simulink model "FILTRO_POTENTE"  (R2020a)
settings: Solver=VariableStepAuto  StartTime=0.0  StopTime=500  RelTol=1e-3
values from neighbouring files (symbols this model uses):
  distanceFromWall = 8    [missionC.m]
  nav_DT = 0.1    [initialization_nav.m]
  nav_giro = 2    [initialization_nav.m]
  nav_h0 = 0    [initialization_nav.m]
  nav_lat0 = cornerC(1)    [initialization_nav.m]
  nav_lon0 = cornerC(2)    [initialization_nav.m]
  nav_plane_AB = coefficient_plane(nav_A,nav_B)    [initialization_nav.m]
  nav_plane_BC = coefficient_plane(nav_B,nav_C)    [initialization_nav.m]
  nav_plane_CD = coefficient_plane(nav_C,nav_D)    [initialization_nav.m]
  nav_plane_DA = coefficient_plane(nav_D,nav_A)    [initialization_nav.m]
undefined symbols (not defined in the file or in its folder): nav_A, nav_B, nav_C, nav_D
(part 3 of 3)

== matlab function FILTRO_POTENTE/Navigation2/Extended Kalman Filter/MISURA VIRTUALE/MATLAB Function ==
  data: x_k_k_1 input; flag_vect input; mis_vect input; e output size=6 1; H output size=6 3; J input; nav_plane_AB parameter; nav_plane_BC parameter; nav_plane_CD parameter; nav_plane_DA parameter
%%
% chiedere ai sensoristi se le posizioni dei sensori equivalgono al centro
% di massa del robot o dobbiamo considerare spostamenti e orientazioni
% relative alla terna body
%%

function [e, H] = virtual(x_k_k_1, flag_vect, mis_vect, J, nav_plane_AB, nav_plane_BC, nav_plane_CD, nav_plane_DA)

    e = zeros(6,1);
    h = zeros(6,1);
    z = zeros(6,1);
    H = zeros(6,3);
    
    
    %valutazione misure GPS
    if mis_vect(3)==1                                   %se i dati del GPS sono validi
        if flag_vect(1) == 1 && flag_vect(2) == 1       %se i dati del GPS sono nuovi
            
            z = z + [mis_vect(1) mis_vect(2) 0 0 0 0]';
            h = h + [x_k_k_1(1)   x_k_k_1(2) 0 0 0 0]';
        
            H(1,:)= [1 0 0];
            H(2,:)= [0 1 0];
        end
    end
    
    %valutazione misure depth
    if flag_vect(4) == 1                                 %se i dati del profondimetro sono nuovi
            
        z = z + [0 0 mis_vect(4) 0 0 0]'; 
        h = h + [0 0  x_k_k_1(3) 0 0 0]';

        H(3,:)= [0 0 1];
    end
    
    %valutiamo ora le misure virtuali solo se quelle del GPS non sono
    %valide
    if mis_vect(3)==0                      %se i dati del GPS non sono validi
        
        if flag_vect(5) == 1               %se i dati del sonar di prua sono nuovi
                
                versore_son_NED = J*[1 0 0]';          %versore terna NED sonar prua
                
                [distanza, plane] = inter(x_k_k_1, versore_son_NED ,nav_plane_AB,nav_plane_BC,nav_plane_CD,nav_plane_DA);
                z = z + [0 0 0 mis_vect(5) 0 0]'; 
                h = h + [0 0 0 distanza    0 0]';
                
                H_new=zeros(1,3);
                [H_new(1), H_new(2), H_new(3)] = calc_H_vect(x_k_k_1, versore_son_NED,plane);
                H(4,:) = H_new;                
        end
    
        if flag_vect(6) == 1               %se i dati del sonar destro sono nuovi
                
                versore_son_NED = J*[0 1 0]';          %versore terna NED sonar dx
                
                [distanza, plane] = inter(x_k_k_1, versore_son_NED ,nav_plane_AB,nav_plane_BC,nav_plane_CD,nav_plane_DA);
                z = z + [0 0 0 0 mis_vect(6) 0]'; 
                h = h + [0 0 0 0 distanza    0]';
                
                H_new=zeros(1,3);
                [H_new(1), H_new(2), H_new(3)] = calc_H_vect(x_k_k_1, versore_son_NED,plane);
                H(5,:) = H_new;
        end
    
        if flag_vect(7) == 1               %se i dati del sonar sinistro sono nuovi
                 
                versore_son_NED = J*[0 -1 0]';          %versore terna NED sonar sx
                
                [distanza, plane] = inter(x_k_k_1, versore_son_NED ,nav_plane_AB,nav_plane_BC,nav_plane_CD,nav_plane_DA);
                z = z + [0 0 0 0 0 mis_vect(7)]'; 
                h = h + [0 0 0 0 0 distanza   ]'; 
                
                H_new=zeros(1,3);
                [H_new(1), H_new(2), H_new(3)] = calc_H_vect(x_k_k_1, versore_son_NED,plane);
                H(6,:) = H_new;
        end
    end
    
    e = z - h;
    
    %%riduco le dimensioni della matrice H e del vettore e
    
    i=0;
    if mis_vect(3) == 0                    %se i dati del GPS non sono validi
        H(1-i,:) = [];
        e(1-i) = [];
        i=i+1;
        H(2-i,:) = [];
        e(2-i) = [];
        i=i+1;
        if flag_vect(4) == 0               %se i dati del profondimetro non sono nuovi
            H(3-i,:) = [];
            e(3-i) = [];
            i=i+1;
        end
        if flag_vect(5) == 0               %se i dati del sonar di prua non sono nuovi
            H(4-i,:) = [];
            e(4-i) = [];
            i=i+1;
        end
        if flag_vect(6) == 0               %se i dati del sonar sinistro non sono nuovi
            H(5-i,:) = [];
            e(5-i) = [];
            i=i+1;
        end
        if flag_vect(7) == 0               %se i dati del sonar destro non sono nuovi
            H(6-i,:) = [];
            e(6-i) = [];
        end
    % da qui invece abbiamo il GPS valido
    else
        if flag_vect(1)==0 || flag_vect(2)==0  %se i dati del GPS non sono nuovi
            H(1-i,:) = [];
            e(1-i) = [];
            i=i+1;
            H(2-i,:) = [];
            e(2-i) = [];
            i=i+1;
        end
        
        if flag_vect(4) == 0               %se i dati del profondimetro non sono nuovi
            H(3-i,:) = [];
            e(3-i) = [];
            i=i+1;
        end
        
        H(4-i,:) = [];                      %annulliamo le misure dei sonar
        e(4-i) = [];
        i=i+1;
        H(5-i,:) = [];
        e(5-i) = [];
        i=i+1;
        H(6-i,:) = [];        
        e(6-i) = [];    
    end
    i=0;
end



%%
%%%%%%%%%%%%%%%%%%%%%%%%%%%%%%%%%%%%%%%%%%%%%%%%%%%%%%%%%%%%%%%%%%%%%%%%%%%%%%%%%%%%%%%%

function [dist, plane] = inter(pos, versore_son_NED,nav_plane_AB,nav_plane_BC,nav_plane_CD,nav_plane_DA)
    
    %calcolo della distanza dalla posizione ai piani delle pareti seguendo
    %la direzione data dal versore del sonar

    t_AB = -(pos(1)+nav_plane_AB(2)*pos(2)+nav_plane_AB(4))/(nav_plane_AB(2)*versore_son_NED(2)+versore_son_NED(1));
    t_BC = -(pos(1)+nav_plane_BC(2)*pos(2)+nav_plane_BC(4))/(nav_plane_BC(2)*versore_son_NED(2)+versore_son_NED(1));
    t_CD = -(pos(1)+nav_plane_CD(2)*pos(2)+nav_plane_CD(4))/(nav_plane_CD(2)*versore_son_NED(2)+versore_son_NED(1));
    t_DA = -(pos(1)+nav_plane_DA(2)*pos(2)+nav_plane_DA(4))/(nav_plane_DA(2)*versore_son_NED(2)+versore_son_NED(1));
    
    if t_AB < 0
        t_AB = inf;
    end
    if t_BC < 0
        t_BC = inf;
    end
    if t_CD < 0
        t_CD = inf;
    end
    if t_DA < 0
        t_DA = inf;
    end
           
    [dist, index] = min([t_AB t_BC t_CD t_DA]);
    dist = dist - 0.267;       %va tolto il raggio del robot rispetto al centro di massa
    
    switch index
        case 1
            plane = nav_plane_AB;
        case 2
            plane = nav_plane_BC;
        case 3
            plane = nav_plane_CD;
        case 4
            plane = nav_plane_DA;
        otherwise
            plane=[0 0 0 0];
            disp('errore nella intersezione del piano')
    end
    
end

function [H1, H2, H3]= calc_H_vect(pos, sonar, plane)

    H1 = sign(pos(1) + plane(4) + pos(2)*plane(2))/abs(sonar(1) + plane(2)*sonar(2));
    H2 = (plane(2)*sign(pos(1) + plane(4) + pos(2)*plane(2)))/abs(sonar(1) + plane(2)*sonar(2));   
    H3 = 0;
end

== matlab function FILTRO_POTENTE/Navigation2/Extended Kalman Filter/PREDIZIONE/Passo di Predizione ==
  data: x0 input; P0 input; x_k_1 input; u_k_1 input; x_k output; P_k_1 input; P_k output size=3 3; J input; L input; Q_k_1 input; nav_DT parameter; nav_flag_init input; nav_flag_init output
%% Passo di PREDIZIONE

function [x_k,  P_k, nav_flag_init] = prediction(x0, P0, x_k_1, u_k_1,  P_k_1, J, L, Q_k_1, nav_DT, nav_flag_init)
    
    x_k = zeros(3,1);
    P_k = zeros(3,3);

    % il valore di nav_flag_init è all'inizio della simulazione pari a 0
    % appena c'è il primo dato disponibile del GPS (insieme al profondimetro)
    % si assume quella come punto di inizializzazione del filtro.

    if nav_flag_init ~= 0      
        if nav_flag_init == 1
            x_k_1 = x0;
            P_k_1 = P0;
            nav_flag_init = 2;      % =2 così l'inizializzazione è fatta una sola volta.
        end
        
        %passo di predizione       
        x_k = x_k_1 + nav_DT*J*u_k_1;
        P_k = P_k_1 + L*Q_k_1*L';               %la matrice F è F = I
           
    end
end

== matlab function FILTRO_POTENTE/Navigation2/Extended Kalman Filter/Q_error/MATLAB Function4 ==
  data: Q input; Q_k_1 input; Q_k output; flag_AHRS input; flag_DVL input
function Q_k = fcn(Q, Q_k_1, flag_AHRS, flag_DVL)

    Q_k = Q;
    
    K=10;
    if flag_DVL == 1
       Q_k = Q_k_1 + K*diag([0,0,0,(0.012)^2,(0.012)^2,(0.012)^2]);
    end
    
    if flag_AHRS == 1
       Q_k = Q_k_1 + K*diag([0.0087, 0.0087, 0.0017,0,0,0]);  
    end
        
end

== matlab function FILTRO_POTENTE/Navigation2/Gyro_check/MATLAB Function4 ==
  data: flag_gyro output; gyro_new input; gyro_now output; gyro_old input
function [flag_gyro, gyro_now] = fcn(gyro_new, gyro_old)

    if isnan(gyro_new(1,1)) || isnan(gyro_new(2,1)) || isnan(gyro_new(3,1))
        gyro_now = gyro_old;
        flag_gyro = 1;
        disp('Misura gyro non valida')
    else
        gyro_now = gyro_new;
        flag_gyro = 0;
    end  
end

== matlab function FILTRO_POTENTE/Navigation2/MATLAB Function ==
  data: u input; y output
function y = Wrap2pi(u)
y = [0;0;0];
coder.extrinsic('wrapToPi');
y = wrapToPi(u);
end

== matlab function FILTRO_POTENTE/Navigation2/MATLAB Function1 ==
  data: u input; dev_standard_xy output; dev_standard_z output
function [dev_standard_xy,dev_standard_z] = fcn(u) 
    
    dev_standard_xy = sqrt(u(1,1)+u(2,2));
    dev_standard_z = sqrt(u(3,3));

end

== matlab function FILTRO_POTENTE/Navigation2/NED2ECEF ==
  data: pos_es_NED input; pos_es_ECEF output; nav_lat0 parameter; nav_lon0 parameter; nav_h0 parameter


function pos_es_ECEF = pos_NED2ECEF(pos_es_NED,nav_lat0, nav_lon0, nav_h0)
     
    coder.extrinsic('evalin', 'wgs84Ellipsoid', 'ned2geodetic');
    pos_es_ECEF = zeros(3,1);
    depth = pos_es_NED(3); 
    
    [pos_es_ECEF(1),pos_es_ECEF(2),pos_es_ECEF(3)]= ned2geodetic(pos_es_NED(1),pos_es_NED(2),0,nav_lat0,nav_lon0,nav_h0,wgs84Ellipsoid);
    pos_es_ECEF(3) = depth;
end

== matlab function FILTRO_POTENTE/Navigation2/SOS_flag_generator/MATLAB Function ==
  data: P_es input; SOS output; DVL input; AHRS input; gyro input; contatore input size=3 1; contatore output
%% Generazione flag di emergenza
% 1. Assenza di segnali dai sensori per un determinato tempo

function [SOS, contatore] = SOS_flag(P_es, DVL, AHRS, gyro, contatore)
    SOS=0;
 
    soglia_P = 10; %[m^2]
    if P_es(1,1)+P_es(2,2) > soglia_P || P_es(3,3) > soglia_P
        SOS=1;
    end
    
    if DVL == 1 
        contatore(1) = contatore(1) + 1;
    else
        contatore(1) = 0;
    end
    
    if AHRS == 1 
        contatore(2) = contatore(2) + 1;
    else
        contatore(2) = 0;
    end
    
    if gyro == 1 
        contatore(3) = contatore(3) + 1;
    else
        contatore(3) = 0;
    end
    
    if max(contatore) > 20
        SOS=1;
    end
    
    

end

== matlab function FILTRO_POTENTE/Navigation1/ECEF2NED ==
  data: GPS_ECEF input; GPS_NED output; nav_lat0 parameter; nav_lon0 parameter; nav_h0 parameter
%Componente di ingresso in terna ECEF
%Lat  [gradi]
%Long  [gradi]
%flag data_valid

function GPS_NED = GPS_conv_valid(GPS_ECEF, nav_lat0, nav_lon0, nav_h0)
    
    coder.extrinsic('evalin', 'wgs84Ellipsoid', 'geodetic2ned');

    if GPS_ECEF(3)==1
        GPS_NED = zeros(3,1);
        [GPS_NED(1),GPS_NED(2),GPS_NED(3)]= geodetic2ned(GPS_ECEF(1),GPS_ECEF(2),0,nav_lat0,nav_lon0,nav_h0,wgs84Ellipsoid);
        GPS_NED(3) = GPS_ECEF(3);
    else                            %qui ci risparmiamo la conversione se il dato non è valido
        GPS_NED = GPS_ECEF; 
    end
end

== matlab function FILTRO_POTENTE/Navigation1/Extended Kalman Filter/CORREZIONE/MATLAB Function ==
  data: x_k_k_1 input; x_k output; P_k_k_1 input; e input size=6 1; H input size=6 3; R_k input size=6 6; P_k output; nav_flag_init input


function [x_k, P_k] = correction(x_k_k_1,P_k_k_1, e, H, R_k,nav_flag_init)
    
     x_k = zeros(3,1);
     P_k = zeros(3,3);
     
     
    if nav_flag_init ~= 0
        %matrice ottenuta da derivata di funzione h (6x1) per i rumori sei vari
        %sensori, che sono 6. (ha dimensione 6x6)
        %andrebbero anche considerati i rumori legati all'AHRS che al momento
        %sono trascurati
        %M = eye(6,6);              %M è l'dientità
        S_k = H*P_k_k_1*H'+ R_k;
        K_k = P_k_k_1*H'*(inv(S_k));

        P_k = (eye(3)-(K_k*H))*P_k_k_1;
        x_k = x_k_k_1 + K_k * e;
    end

end

== matlab function FILTRO_POTENTE/MATLAB Function ==
  data: u input; y output
function y = fcn(u)
u(3)=1;
y = u;

== matlab function FILTRO_POTENTE/Navigation1/Extended Kalman Filter/Creazione vettore delle misure ==
  data: flag_vect output; GPS input; mis_vect output; depth input; s_pr input; s_dx input; s_sx input; mis_vect_prec input; J input; pos input; nav_plane_AB parameter; nav_plane_BC parameter; nav_plane_CD parameter; nav_plane_DA parameter; nav_A parameter; nav_B parameter; nav_C parameter; nav_D parameter; distanceFromWall parameter
%%
% Questa funzione impila le informazioni derivanti dai vari sensori in un
% unico vettore mis_vect 7x1.                                 
% Ci sarà un corrispondente vettore flag_vect 7x1 di flag che sarà pari a:

% flag(i) = 0  se la misura è uguale a quella arrivata nell'istante
% predecente, in tal caso la correzione non verrà effettuata
% flag(i) = 1 se la misura è stata aggiornata rispetto a quella precendente
 
% NB il controllo sulla validità dei dati del GPS è valutata nel blocco
% sucessivo

function [flag_vect,mis_vect] = misure_vector(GPS,depth,s_pr,s_dx,s_sx, mis_vect_prec,...
          J,pos, nav_plane_AB, nav_plane_BC, nav_plane_CD, nav_plane_DA, nav_A, nav_B, nav_C, nav_D, distanceFromWall)
    
    mis_vect = zeros(7,1);
    flag_vect = zeros(7,1);
	mis_vect = [GPS(1) GPS(2) GPS(3) depth s_pr s_dx s_sx]';
    
    for i=[1:7]
        if mis_vect(i) ~= mis_vect_prec(i)
            flag_vect(i) = 1;
        end
    end
    
    %valutiamo se la misura del profondimetro è valida
    if isnan(depth)  
        flag_vect(4) = 0;
    end
     
    %se i dati dei sonar qui sono utilizzabili, dobbiamo assicurarci che il 
    %loro raggio non punti verso uno spigolo, in quel caso potrebbe
    %causare una correzione errata
    
    if flag_vect(5) == 1               %se i dati del sonar di prua sono nuovi
            versore_son_NED = J*[1 0 0]';          %versore terna NED sonar prua
            flag_vect(5) = inter(pos, versore_son_NED ,nav_plane_AB,nav_plane_BC,nav_plane_CD,nav_plane_DA, nav_A, nav_B, nav_C, nav_D);       
    end

    if flag_vect(6) == 1               %se i dati del sonar destro sono nuovi
            versore_son_NED = J*[0 1 0]';          %versore terna NED sonar dx

            flag_vect(6) = inter(pos, versore_son_NED ,nav_plane_AB,nav_plane_BC,nav_plane_CD,nav_plane_DA, nav_A, nav_B, nav_C, nav_D);       
    end
    if flag_vect(7) == 1               %se i dati del sonar sinistro sono nuovi
            versore_son_NED = J*[0 -1 0]';          %versore terna NED sonar sx
            flag_vect(7) = inter(pos, versore_son_NED ,nav_plane_AB,nav_plane_BC,nav_plane_CD,nav_plane_DA, nav_A, nav_B, nav_C, nav_D);
    end 
    %la terza componente di flag_vect non sarà utilizzata. per assicurarci
    %che i dati del GPS siano validi ci rifaremo sempre su mis_vect
    
    
    
    %se il valore del sonar è NaN, non dobbiamo considerare valide le
    %misure, e se il robot troppo lontane dalle pareti
    soglia_distanza=distanceFromWall*3;
    soglia_variazione=0.8;
    if isnan(s_pr) || mis_vect(5) > soglia_distanza || abs(mis_vect(5)- mis_vect_prec(5)) > soglia_variazione
        flag_vect(5) = 0;
    end
    if isnan(s_dx) || mis_vect(6) > soglia_distanza || abs(mis_vect(6)- mis_vect_prec(6)) > soglia_variazione
        flag_vect(6) = 0;
    end
    if isnan(s_sx) || mis_vect(7) > soglia_distanza || abs(mis_vect(7)- mis_vect_prec(7)) > soglia_variazione
        flag_vect(7) = 0;
    end
end




function [flag] = inter(pos, versore_son_NED,nav_plane_AB,nav_plane_BC,nav_plane_CD,nav_plane_DA, nav_A, nav_B, nav_C, nav_D)
    
    %calcolo della distanza dalla posizione ai piani delle pareti seguendo
    %la direzione data dal versore del sonar

    t_AB = -(pos(1)+nav_plane_AB(2)*pos(2)+nav_plane_AB(4))/(nav_plane_AB(2)*versore_son_NED(2)+versore_son_NED(1));
    t_BC = -(pos(1)+nav_plane_BC(2)*pos(2)+nav_plane_BC(4))/(nav_plane_BC(2)*versore_son_NED(2)+versore_son_NED(1));
    t_CD = -(pos(1)+nav_plane_CD(2)*pos(2)+nav_plane_CD(4))/(nav_plane_CD(2)*versore_son_NED(2)+versore_son_NED(1));
    t_DA = -(pos(1)+nav_plane_DA(2)*pos(2)+nav_plane_DA(4))/(nav_plane_DA(2)*versore_son_NED(2)+versore_son_NED(1));
    
    if t_AB < 0
        t_AB = inf;
    end
    if t_BC < 0
        t_BC = inf;
    end
    if t_CD < 0
        t_CD = inf;
    end
    if t_DA < 0
        t_DA = inf;
    end
           
    [dist, index] = min([t_AB t_BC t_CD t_DA]);
    dist = dist - 0.267;       %va tolto il raggio del robot rispetto al centro di massa
    
    int=zeros(1,3);
    %calcolo l'intersezione
    int(1) = pos(1) + versore_son_NED(1)*dist;
    int(2) = pos(2) + versore_son_NED(2)*dist;
    int(3) = 0;
    
    
    
    soglia_spigolo = 5;          %distanza massima dallo spigolo entro la quale 
                       %la misura del sonar non è buona
    flag=1;
    switch index
        case 1      
            if norm(int-nav_A) < soglia_spigolo || norm(int-nav_B) < soglia_spigolo
                flag=0;
            end
        case 2
            if norm(int-nav_B) < soglia_spigolo || norm(int-nav_C) < soglia_spigolo
                flag=0;
            end
        case 3
            if norm(int-nav_C) < soglia_spigolo || norm(int-nav_D) < soglia_spigolo
                flag=0;
            end
        case 4
            if norm(int-nav_D) < soglia_spigolo || norm(int-nav_A) < soglia_spigolo
                flag=0;
            end
        otherwise
            disp('errore nella intersezione del piano')
    end
end
